simulink model "untitled"  (R2018a)
settings: Solver=FixedStepDiscrete  StartTime=0.0  StopTime=20  FixedStep=1e-6  RelTol=1e-3
libraries: dspadpt3 x1
settings Model: Creator=ljs  LastModifiedBy=ljs

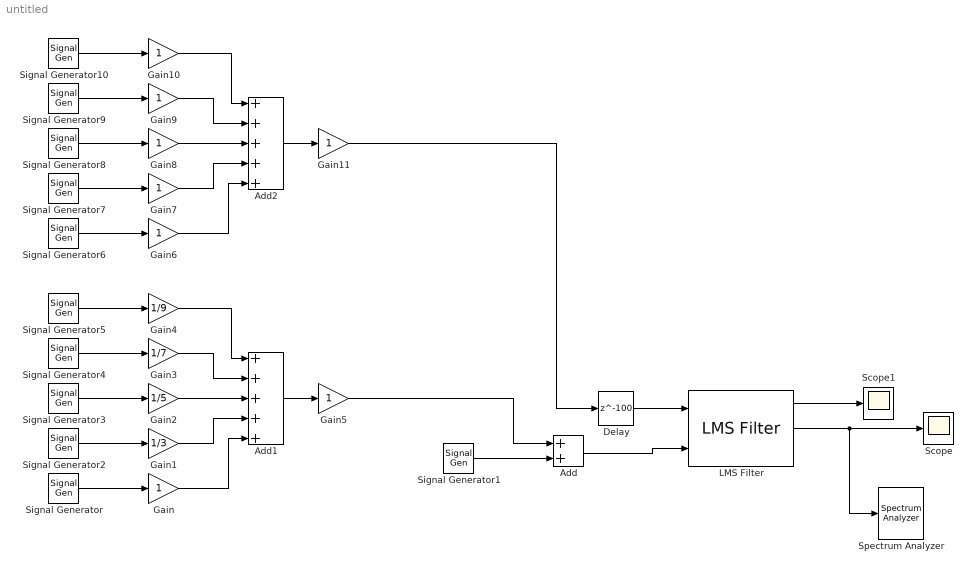
== system untitled ==
  Add : Sum
  Add1 : Sum  Inputs=5
  Add2 : Sum  Inputs=5
  Delay : Delay  DelayLength=100
  Gain{,5..11} (8 alike) : Gain
  Gain1 : Gain  Gain=1/3
  Gain2 : Gain  Gain=1/5
  Gain3 : Gain  Gain=1/7
  Gain4 : Gain  Gain=1/9
  LMS Filter : dspadpt3/LMS Filter  Algo=LMS  L=128*3  stepflag=Dialog  mu=0.00000001  leakage=1.0  ic=0  Adapt=off  resetflag=None  weights=on  secondCoeffMode=User-defined  secondCoeffWordLength=2  secondCoeffFracLength=15  accum2Mode=User-defined  accum2FracLength=20  prodOutput2Mode=User-defined  prodOutput2FracLength=20  prodOutput3Mode=User-defined  prodOutput3FracLength=20  prodOutput4Mode=User-defined  prodOutput4FracLength=20  quotientMode=User-defined  quotientFracLength=20  roundingMode=Floor  overflowMode=off  addnparflag=off
      settings: SourceProductName=DSP System Toolbox  SourceProductBaseCode=DS
  Scope : Scope
  Scope1 : Scope
  Signal Generator : SignalGenerator  Frequency=10e3
  Signal Generator1 : SignalGenerator  Frequency=30e3+10
  Signal Generator10 : SignalGenerator  Frequency=90e3
  Signal Generator2 : SignalGenerator  Frequency=30e3
  Signal Generator3 : SignalGenerator  Frequency=50e3
  Signal Generator4 : SignalGenerator  Frequency=70e3
  Signal Generator5 : SignalGenerator  Frequency=90e3
  Signal Generator6 : SignalGenerator  Frequency=10e3
  Signal Generator7 : SignalGenerator  Frequency=30e3
  Signal Generator8 : SignalGenerator  Frequency=50e3
  Signal Generator9 : SignalGenerator  Frequency=70e3
  Spectrum Analyzer : SpectrumAnalyzer
  wires:
  Add/1 -> LMS Filter/2
  Signal Generator1/1 -> Add/2
  Delay/1 -> LMS Filter/1
  LMS Filter/1 -> Scope1/1
  LMS Filter/2 -> Spectrum Analyzer/1, Scope/1
  Signal Generator5/1 -> Gain4/1
  Signal Generator4/1 -> Gain3/1
  Signal Generator3/1 -> Gain2/1
  Signal Generator2/1 -> Gain1/1
  Signal Generator/1 -> Gain/1
  Gain2/1 -> Add1/3
  Gain3/1 -> Add1/2
  Gain4/1 -> Add1/1
  Gain1/1 -> Add1/4
  Gain/1 -> Add1/5
  Add1/1 -> Gain5/1
  Gain5/1 -> Add/1
  Signal Generator7/1 -> Gain7/1
  Signal Generator9/1 -> Gain9/1
  Gain6/1 -> Add2/5
  Signal Generator6/1 -> Gain6/1
  Gain9/1 -> Add2/2
  Gain10/1 -> Add2/1
  Signal Generator8/1 -> Gain8/1
  Gain8/1 -> Add2/3
  Signal Generator10/1 -> Gain10/1
  Gain7/1 -> Add2/4
  Add2/1 -> Gain11/1
  Gain11/1 -> Delay/1
